simulink model "mymodel_sim"  (R2019b)
settings: Solver=VariableStepAuto  StartTime=0.0  StopTime=20  RelTol=1e-3
values from neighbouring files (symbols this model uses):
  stepf = 1    [MainScript.m]
  stepi = 0    [MainScript.m]
  stept = 2    [MainScript.m]
  tau = 0.5    [MainScript.m]
  x0 = 0    [MainScript.m]
settings Model: Creator=mountj  LastModifiedBy=n9182250
settings DataIOCC: TimeSaveName=mytime

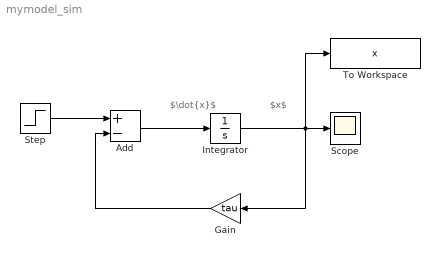
== system mymodel_sim ==
  note: $\dot{x}$
  note: $x$
  Add : Sum  Inputs=+-
  Gain : Gain  Gain=tau
  Integrator : Integrator  InitialCondition=x0
  Scope : Scope
  Step : Step  Time=stept  Before=stepi  After=stepf  SampleTime=0
  To Workspace : ToWorkspace  VariableName=x  SampleTime=-1
  wires:
  Step/1 -> Add/1
  Add/1 -> Integrator/1
  Integrator/1 -> Gain/1, Scope/1, To Workspace/1
  Gain/1 -> Add/2
